simulink model "Helicopter_Model_Draft"  (R2024b)
settings: Solver=VariableStepAuto  StartTime=0.0  StopTime=100.0  RelTol=1e-3
StartFcn:
  | L1 = 3.13;
undefined symbols (not defined in the file): Earth, gravity, hRef, rad, rho, s, VRef, WGS84
libraries: slpidlib x9, simulink x2, aerolibfltsims x2, matrix_library x2, aerolibconvert2 x2, aerolibsim3d x2, aerolibatmos2 x1, aerolibtransform2 x1, shared6dof x1, sim3dlib x1
(part 2 of 2)

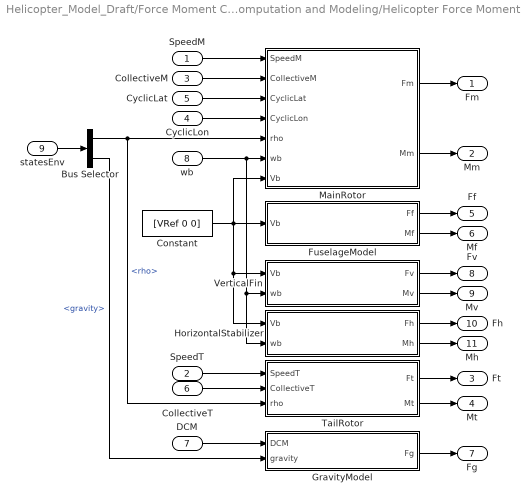
== system Helicopter_Model_Draft/Force Moment Computation and Modeling/Helicopter Force Moment Computation/ComputeForceandMoment ==
  SpeedM : Inport
  SpeedT : Inport  Port=2
  CollectiveM : Inport  Port=3
  CyclicLon : Inport  Port=4
  CyclicLat : Inport  Port=5
  CollectiveT : Inport  Port=6
  DCM : Inport  Port=7
  wb : Inport  Port=8
  statesEnv : Inport  Port=9
  Bus Selector : BusSelector  OutputSignals=rho,gravity
  Constant : Constant  Value=[VRef 0 0]
  FuselageModel : Subsystem
  GravityModel : Subsystem
  HorizontalStabilizer : MATLAB Function  TreatAsAtomicUnit=on
  MainRotor : Subsystem
  TailRotor : Subsystem
  VerticalFin : MATLAB Function  TreatAsAtomicUnit=on
  Fm : Outport
  Mm : Outport  Port=2
  Ft : Outport  Port=3
  Mt : Outport  Port=4
  Ff : Outport  Port=5
  Mf : Outport  Port=6
  Fg : Outport  Port=7
  Fv : Outport  Port=8
  Mv : Outport  Port=9
  Fh : Outport  Port=10
  Mh : Outport  Port=11
  wires:
  TailRotor/2(Mt) -> Mt/1
  MainRotor/1(Fm) -> Fm/1
  TailRotor/1(Ft) -> Ft/1
  FuselageModel/1(Ff) -> Ff/1
  MainRotor/2(Mm) -> Mm/1
  FuselageModel/2(Mf) -> Mf/1
  GravityModel/1(Fg) -> Fg/1
  Constant/1 -> HorizontalStabilizer/1(Vb), VerticalFin/1(Vb), MainRotor/7(Vb), FuselageModel/1(Vb)
  SpeedM/1 -> MainRotor/1(SpeedM)
  CollectiveT/1 -> TailRotor/2(CollectiveT)
  CollectiveM/1 -> MainRotor/2(CollectiveM)
  SpeedT/1 -> TailRotor/1(SpeedT)
  VerticalFin/1(Fv) -> Fv/1
  VerticalFin/2(Mv) -> Mv/1
  HorizontalStabilizer/1(Fh) -> Fh/1
  HorizontalStabilizer/2(Mh) -> Mh/1
  DCM/1 -> GravityModel/1(DCM)
  CyclicLon/1 -> MainRotor/4(CyclicLon)
  CyclicLat/1 -> MainRotor/3(CyclicLat)
  wb/1 -> HorizontalStabilizer/2(wb), VerticalFin/2(wb), MainRotor/6(wb)
  statesEnv/1 -> Bus Selector/1
  Bus Selector/1 -> MainRotor/5(rho), TailRotor/3(rho)  "<rho>"
  Bus Selector/2 -> GravityModel/2(gravity)  "<gravity>"

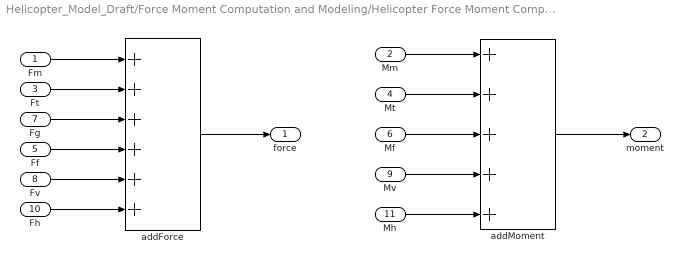
== system Helicopter_Model_Draft/Force Moment Computation and Modeling/Helicopter Force Moment Computation/ResultantForcesandMoments ==
  Fm : Inport
  Mm : Inport  Port=2
  Ft : Inport  Port=3
  Mt : Inport  Port=4
  Ff : Inport  Port=5
  Mf : Inport  Port=6
  Fg : Inport  Port=7
  Fv : Inport  Port=8
  Mv : Inport  Port=9
  Fh : Inport  Port=10
  Mh : Inport  Port=11
  addForce : Sum  Inputs=++++++
  addMoment : Sum  Inputs=+++++
  force : Outport
  moment : Outport  Port=2
  wires:
  Mt/1 -> addMoment/2
  Mf/1 -> addMoment/3
  addMoment/1 -> moment/1
  Ft/1 -> addForce/2
  Fm/1 -> addForce/1
  Fg/1 -> addForce/3
  Mm/1 -> addMoment/1
  Ff/1 -> addForce/4
  addForce/1 -> force/1
  Mh/1 -> addMoment/5
  Fh/1 -> addForce/6
  Fv/1 -> addForce/5
  Mv/1 -> addMoment/4

== system Helicopter_Model_Draft/Visualization/Variant Subsystem/Scope Visualization ==
  states : Inport
  Bus Selector : BusSelector  OutputSignals=Xe,angles,Vb,wb
  angle : Scope
  position : Scope
  rates : Scope
  velocity : Scope
  wires:
  states/1 -> Bus Selector/1
  Bus Selector/1 -> position/1  "<Xe>"
  Bus Selector/4 -> rates/1  "<wb>"
  Bus Selector/3 -> velocity/1  "<Vb>"
  Bus Selector/2 -> angle/1  "<angles>"

== system Helicopter_Model_Draft/Visualization/Variant Subsystem/Simulink 3D Animation ==
  states : Inport
  Add : Sum
  Bus Selector : BusSelector  OutputSignals=Xe,angles
  Constant10 : Constant  Value=[5000 0 -0.06]  VectorParams1D=off
  Simulation 3D Light Helicopter Pack : aerolibsim3d/Simulation 3D Light Helicopter Pack  Engine_T=off  Engine_R=off  Rotor1_T=off  Rotor1_R=on  Rotor2_T=off  Rotor2_R=on  Sensor1_T=off  Sensor1_R=off  Sensor2_T=off  Sensor2_R=off  GeoRadioButton=NED  AdjustForCesium=off  Heading0=90
  Simulation 3D Rotorcraft : aerolibsim3d/Simulation 3D Rotorcraft  Priority=-1  Mesh=Light helicopter  MeshPath=/MathWorksAerospaceContent/Vehicles/Rotorcraft/Helicopter/Mesh/SK_Helicopter.SK_Helicopter  MeshPathLight=/MathWorksAerospaceContent/Vehicles/Rotorcraft/LightHelicopter/Mesh/SK_LightHelicopter.SK_LightHelicopter  MeshPathMulti=/MathWorksAerospaceContent/Vehicles/Rotorcraft/Multirotor/Mesh/SK_Quadcopter.SK_Quadcopter  AircraftColor=Red  ActorName=SimulinkVehicle1  Translation=[5000 0 -0.06;zeros(5,3)]  Rotation=zeros(6, 3)  ScaleInputPort=Dialog  Scale=[1 1 1]  InitialScale=[1 1 1]  IsGHSensorEnabled=off  AreGHRaysVisible=off  IsOutputReshapeEnabled=off  GHRayLength=1524  GHBodyOffset=1.169  GHFrontTireRadius=0.196  GHLeftTireRadius=0.203  GHRightTireRadius=0.203  GHContactLocation1=[1.47 -1.04 1.169]  GHContactLocation2=[-1.24 -1.04 1.169]  GHContactLocation3=[-1.24 1.04 1.169]  GHContactLocation4=[1.47 1.04 1.169]  WoWSensorTolerance=0.05  LightsConfig=Automatic lights  LandingLightIntensity=300000  LandingLightConeAngle=15  LandingLightColor=[1 1 1]  HelicopterLeftLandingLightLocation=[0 0 0]  HelicopterLeftLandingLightOrientation=[0 0 0]  NoseLightIntensity=150000  NoseLightConeAngle=36  HelicopterNoseLightLocation=[0 0 0]  HelicopterNoseLightOrientation=[0 0 0]  NavLightIntensity=500  PositionLightIntensity=500  StrobeLightIntensity=5000  StrobeLightColor=[1 1 1]  StrobePeriod=1.5  StrobePulseWidth=6  BeaconLightIntensity=4000  BeaconLightColor=[1 0 0]  BeaconPeriod=1.5  BeaconPulseWidth=10  SampleTime=-1  ActorType=SimulinkVehicle  ID=1  aMode=0  ActorTag=SimulinkVehicle1
  Simulation 3D Scene Configuration : sim3dlib/Simulation 3D Scene Configuration  Priority=0  ProjectFormat=Default Scenes  SceneDesc=Airport  ProjectName=C:\Program Files\MATLAB\R2024b\toolbox\shared\sim3d_projects\automotive_project_windows\UE\WindowsNoEditor\VehicleSimulation.exe  ScenePath=/Game/Maps/HwStrght  EnableOpenDRIVE=off  vehTagList={'Scene Origin';'SimulinkVehicle1'}  vehTag=SimulinkVehicle1  FreeCameraInitialTranslation=[-6, 0, 2]  FreeCameraDefaultInitialTranslation=[-6, 0, 2]  FreeCameraInitialRotation=[0, -15, 0]  FreeCameraDefaultInitialRotation=[0, -15, 0]  OpVisEn=off  Ts=.02  EnableWindow=on  EnableRemoteAccess=off  EnableWeather=off  SunAzimuth=90  SunAltitude=40.0  EnableGeospatialSun=off  Latitude=0  Longitude=0  Date=2023-01-01  Time=10:30:00  GeoTimeZone=-5.0  SunDaylightSaving=off  wind=1  clouds=10  EnableVolumetricClouds=off  CloudCoverage=0  CloudAltitude=6  fog=0  rain=0  RaindropsEffect=off  SnowDensity=0  EnableGeospatial=off  UseTrueOrigin=off  OriginHeight=200  OriginLatitude=40.744652  OriginLongitude=-73.988864  MapStyle=Aerial  AdditionalAssetIDs=[]  UseAdvancedSunSky=off  SolarTime=11  TimeZone=-5  Day=21  Month=9  Year=2022  UseDaylightSavingTime=on  DSTStartDay=10  DSTStartMonth=3  DSTEndDay=3  DSTEndMonth=11  DSTSwitchHour=2  sensorTag=MainCamera1  sensorId=1  sensorName=MainCamera1  mountLoc=Origin  offsetFlag=off  tmountOffset=[0, 0, 0]  rmountOffset=[0, 0, 0]  HorizontalResolution=1280  VerticalResolution=720  HorizontalFOV=60  mountPoint=[0 0 0]  mountOrientation=[0 0 0]  aMode=0  ID=1  GeoTrigger=Inactive
  Subsystem : Subsystem
  speedM : Constant  Value=34
  speedT : Constant  Value=116
  wires:
  Bus Selector/2 -> Simulation 3D Light Helicopter Pack/2  "<angles>"
  states/1 -> Bus Selector/1
  speedT/1 -> Subsystem/2(SpeedT)
  speedM/1 -> Subsystem/1(SpeedM)
  Simulation 3D Light Helicopter Pack/1 -> Simulation 3D Rotorcraft/1
  Add/1 -> Simulation 3D Light Helicopter Pack/1
  Subsystem/2(Position Blade 2) -> Simulation 3D Light Helicopter Pack/4
  Constant10/1 -> Add/1
  Simulation 3D Light Helicopter Pack/2 -> Simulation 3D Rotorcraft/2
  Subsystem/1(Position Blade1) -> Simulation 3D Light Helicopter Pack/3
  Bus Selector/1 -> Add/2  "<Xe>"

== system Helicopter_Model_Draft/Attitude and Altitude Control/Reference Atttiude and Altitude Definition/Variant Subsystem/Hover ==
  Constant : Constant  Value=0
  ub : Outport
  wires:
  Constant/1 -> ub/1

== system Helicopter_Model_Draft/Attitude and Altitude Control/Reference Atttiude and Altitude Definition/Variant Subsystem/Level ==
  Vb : Inport
  Demux : Demux  Outputs=3
  Saturation1 : Saturate  UpperLimit=65  LowerLimit=0
  Sqrt : Sqrt
  Square1 : Math  Operator=square
  Square2 : Math  Operator=square
  Sum : Sum  Inputs=|+-
  Terminator : Terminator
  Terminator1 : Terminator
  V : Constant  Value=VRef
  ub : Outport
  wires:
  Square2/1 -> Sum/2
  Sum/1 -> Sqrt/1
  Square1/1 -> Sum/1
  Sqrt/1 -> Saturation1/1
  Vb/1 -> Demux/1
  Saturation1/1 -> ub/1
  Demux/3 -> Square2/1
  V/1 -> Square1/1
  Demux/1 -> Terminator/1
  Demux/2 -> Terminator1/1

== system Helicopter_Model_Draft/Force Moment Computation and Modeling/Helicopter Force Moment Computation/ComputeForceandMoment/FuselageModel ==
  Vb : Inport
  Abs : Abs  SaturateOnIntegerOverflow=off
  Abs1 : Abs  SaturateOnIntegerOverflow=off
  Abs2 : Abs  SaturateOnIntegerOverflow=off
  Demux : Demux  Outputs=3
  Fuselage Force Computation : Subsystem
  Fuselage Moment Computation : Subsystem
  Ff : Outport
  Mf : Outport  Port=2
  wires:
  Demux/1 -> Fuselage Force Computation/1(u), Fuselage Moment Computation/1(u), Abs/1
  Demux/2 -> Fuselage Force Computation/3(v), Abs1/1, Fuselage Moment Computation/3(v)
  Demux/3 -> Fuselage Moment Computation/4(w), Abs2/1, Fuselage Force Computation/5(w)
  Abs/1 -> Fuselage Moment Computation/2(absu), Fuselage Force Computation/2(absu)
  Vb/1 -> Demux/1
  Fuselage Moment Computation/1(Mf) -> Mf/1
  Abs1/1 -> Fuselage Force Computation/4(absv)
  Abs2/1 -> Fuselage Force Computation/6(absw)
  Fuselage Force Computation/1(Ff) -> Ff/1

== system Helicopter_Model_Draft/Force Moment Computation and Modeling/Helicopter Force Moment Computation/ComputeForceandMoment/GravityModel ==
  DCM : Inport
  gravity : Inport  Port=2
  Product : Product  Multiplication=Matrix(*)
  mass : Gain  Gain=2800
  Fg : Outport
  wires:
  mass/1 -> Product/2  "Fg_NED"
  gravity/1 -> mass/1
  Product/1 -> Fg/1
  DCM/1 -> Product/1

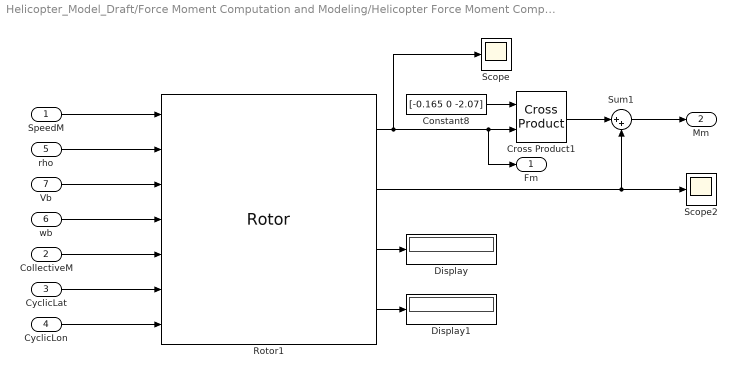
== system Helicopter_Model_Draft/Force Moment Computation and Modeling/Helicopter Force Moment Computation/ComputeForceandMoment/MainRotor ==
  SpeedM : Inport
  CollectiveM : Inport  Port=2
  CyclicLat : Inport  Port=3
  CyclicLon : Inport  Port=4
  rho : Inport  Port=5
  wb : Inport  Port=6
  Vb : Inport  Port=7
  Constant8 : Constant  Value=[-0.165 0 -2.07]  VectorParams1D=off
  Cross Product1 : matrix_library/Cross Product
  Display : Display
  Display1 : Display
  Rotor1 : Rotor  modelMode=With flap effects  controlInput=on  CTCQMode=Compute using BEMT  CT=0.0042  CQ=24e-5  CTout=on  radius=7.35  chord=0.53  cd0=0.009  gamma=10  thetaRoot=0.1493  thetaTwist=-0.1745
  Scope : Scope
  Scope2 : Scope
  Sum1 : Sum  Inputs=|++
  Fm : Outport
  Mm : Outport  Port=2
  wires:
  SpeedM/1 -> Rotor1/1
  Cross Product1/1 -> Sum1/1
  Constant8/1 -> Cross Product1/1
  Sum1/1 -> Mm/1
  Rotor1/2 -> Scope2/1, Sum1/2
  rho/1 -> Rotor1/2
  CollectiveM/1 -> Rotor1/5
  Rotor1/3 -> Display/1
  Rotor1/4 -> Display1/1
  Rotor1/1 -> Scope/1, Fm/1, Cross Product1/2
  wb/1 -> Rotor1/4
  Vb/1 -> Rotor1/3
  CyclicLat/1 -> Rotor1/6
  CyclicLon/1 -> Rotor1/7

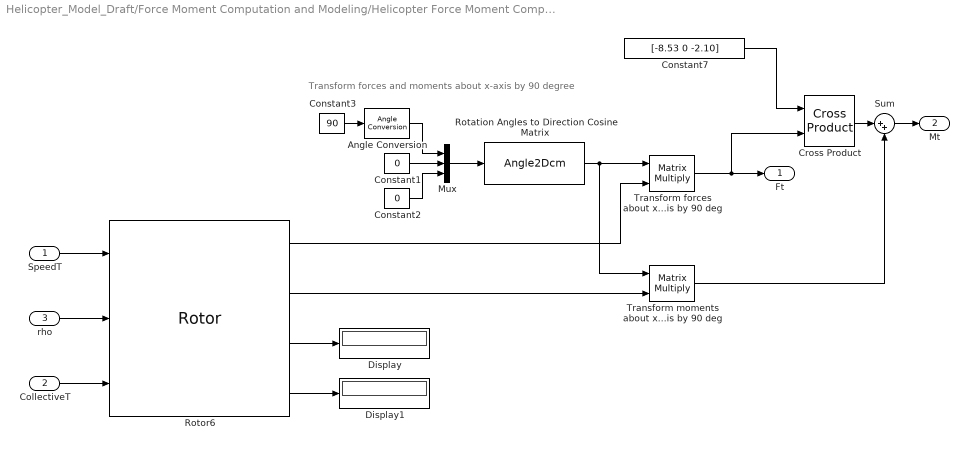
== system Helicopter_Model_Draft/Force Moment Computation and Modeling/Helicopter Force Moment Computation/ComputeForceandMoment/TailRotor ==
  note: Transform forces and moments about x-axis by 90 degree
  SpeedT : Inport
  CollectiveT : Inport  Port=2
  rho : Inport  Port=3
  Angle Conversion : aerolibconvert2/Angle Conversion  IU=deg  OU=rad
  Constant1 : Constant  Value=0
  Constant2 : Constant  Value=0
  Constant3 : Constant  Value=90
  Constant7 : Constant  Value=[-8.53 0 -2.10]  VectorParams1D=off
  Cross Product : matrix_library/Cross Product
  Display : Display
  Display1 : Display
  Mux : Mux  Inputs=3
  Rotation Angles to Direction Cosine Matrix : Angle2Dcm  rotationOrder=XYZ
      settings: AttributesFormatString=Rotation Order: %<rotationOrder>
  Rotor6 : Rotor  controlInput=on  CTCQMode=Compute using BEMT  CTout=on  radius=1.29  chord=0.2133  cd0=0.002  thetaRoot=0.015  thetaTwist=0
  Sum : Sum  Inputs=|++
  "Transform forces about x-axis by 90 deg " : Product  Multiplication=Matrix(*)
  Transform moments about x-axis by 90 deg : Product  Multiplication=Matrix(*)
  Ft : Outport
  Mt : Outport  Port=2
  wires:
  "Transform forces about x-axis by 90 deg "/1 -> Ft/1, Cross Product/2
  Rotor6/1 -> "Transform forces about x-axis by 90 deg "/2
  Transform moments about x-axis by 90 deg/1 -> Sum/2
  SpeedT/1 -> Rotor6/1
  Rotor6/2 -> Transform moments about x-axis by 90 deg/2
  Rotation Angles to Direction Cosine Matrix/1 -> "Transform forces about x-axis by 90 deg "/1, Transform moments about x-axis by 90 deg/1
  Cross Product/1 -> Sum/1
  Constant7/1 -> Cross Product/1
  Sum/1 -> Mt/1
  CollectiveT/1 -> Rotor6/3
  rho/1 -> Rotor6/2
  Rotor6/4 -> Display1/1
  Rotor6/3 -> Display/1
  Angle Conversion/1 -> Mux/1
  Mux/1 -> Rotation Angles to Direction Cosine Matrix/1
  Constant3/1 -> Angle Conversion/1
  Constant1/1 -> Mux/2
  Constant2/1 -> Mux/3

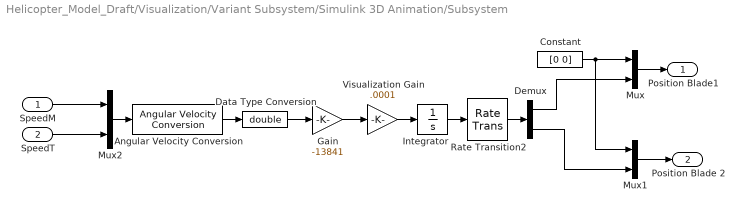
== system Helicopter_Model_Draft/Visualization/Variant Subsystem/Simulink 3D Animation/Subsystem ==
  SpeedM : Inport
  SpeedT : Inport  Port=2
  Angular Velocity Conversion : aerolibconvert2/Angular Velocity Conversion  IU=rad/s  OU=rpm
  Constant : Constant  Value=[0 0]  VectorParams1D=off
  Data Type Conversion : DataTypeConversion  OutDataTypeStr=double  SaturateOnIntegerOverflow=off  RndMeth=Floor
  Demux : Demux  Outputs=2
  Gain : Gain  Gain=-13841
  Integrator : Integrator  InitialCondition="[.1  .1]"  WrapState=on  WrappedStateUpperValue=2*pi  WrappedStateLowerValue=-2*pi
  Mux : Mux  Inputs=2
  Mux1 : Mux  Inputs=2
  Mux2 : Mux  Inputs=2
  Rate Transition2 : RateTransition
  Visualization Gain : Gain  Gain=.0001
  Position Blade1 : Outport  VectorParamsAs1DForOutWhenUnconnected=off
  Position Blade 2 : Outport  Port=2  VectorParamsAs1DForOutWhenUnconnected=off
  wires:
  Demux/2 -> Mux1/2
  Visualization Gain/1 -> Integrator/1
  Constant/1 -> Mux1/1, Mux/1
  Mux1/1 -> Position Blade 2/1
  Data Type Conversion/1 -> Gain/1
  Integrator/1 -> Rate Transition2/1
  Mux/1 -> Position Blade1/1
  Gain/1 -> Visualization Gain/1
  Demux/1 -> Mux/2
  Mux2/1 -> Angular Velocity Conversion/1
  Rate Transition2/1 -> Demux/1
  SpeedM/1 -> Mux2/1
  SpeedT/1 -> Mux2/2
  Angular Velocity Conversion/1 -> Data Type Conversion/1

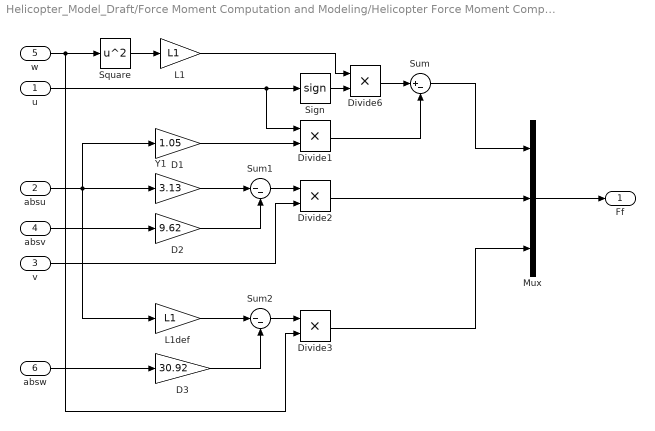
== system Helicopter_Model_Draft/Force Moment Computation and Modeling/Helicopter Force Moment Computation/ComputeForceandMoment/FuselageModel/Fuselage Force Computation ==
  u : Inport
  absu : Inport  Port=2
  v : Inport  Port=3
  absv : Inport  Port=4
  w : Inport  Port=5
  absw : Inport  Port=6
  D1 : Gain  Gain=1.05
  D2 : Gain  Gain=9.62
  D3 : Gain  Gain=30.92
  Divide{1..3,6} (4 alike) : Product  Inputs=**
  L1 : Gain  Gain=L1
  L1def : Gain  Gain=L1
  Mux : Mux  Inputs=3
  Sign : Signum
  Square : Math  Operator=square
  Sum : Sum  Inputs=|+-
  Sum1 : Sum  Inputs=|--
  Sum2 : Sum  Inputs=|--
  Y1 : Gain  Gain=3.13
  Ff : Outport
  wires:
  Sign/1 -> Divide6/2
  D2/1 -> Sum1/2
  Sum1/1 -> Divide2/1
  Divide6/1 -> Sum/1
  Divide2/1 -> Mux/2
  D3/1 -> Sum2/2
  u/1 -> Divide1/1, Sign/1
  L1def/1 -> Sum2/1
  Divide1/1 -> Sum/2
  Y1/1 -> Sum1/1
  absv/1 -> D2/1
  Square/1 -> L1/1
  L1/1 -> Divide6/1
  Sum/1 -> Mux/1
  Divide3/1 -> Mux/3
  Sum2/1 -> Divide3/1
  v/1 -> Divide2/2
  absw/1 -> D3/1
  Mux/1 -> Ff/1
  w/1 -> Square/1, Divide3/2
  absu/1 -> D1/1, Y1/1, L1def/1
  D1/1 -> Divide1/2

== system Helicopter_Model_Draft/Force Moment Computation and Modeling/Helicopter Force Moment Computation/ComputeForceandMoment/FuselageModel/Fuselage Moment Computation ==
  u : Inport
  absu : Inport  Port=2
  v : Inport  Port=3
  w : Inport  Port=4
  Constant : Constant  Value=0
  Divide4 : Product  Inputs=**
  Divide5 : Product  Inputs=**
  M1 : Gain  Gain=13.95
  Mux1 : Mux  Inputs=3
  N1 : Gain  Gain=13.95
  Unary Minus : UnaryMinus
  Mf : Outport
  wires:
  u/1 -> Divide5/1
  M1/1 -> Divide4/2
  N1/1 -> Unary Minus/1
  Mux1/1 -> Mf/1
  Divide5/1 -> Mux1/3
  Constant/1 -> Mux1/1
  v/1 -> N1/1
  Unary Minus/1 -> Divide5/2
  Divide4/1 -> Mux1/2
  w/1 -> M1/1
  absu/1 -> Divide4/1

== matlab function Helicopter_Model_Draft/Force Moment Computation and Modeling/Helicopter Force Moment Computation/ComputeForceandMoment/VerticalFin ==
  data: Vb input; Fv output; wb input; Mv output
function [Fv,Mv] = VerticalFin(Vb,wb)
lvf = 7.62;
K1 = 1.40;
F1 = 0.77;
vf = -Vb(2)+lvf*wb(3);
Yv = K1*vf*Vb(1)+F1*vf*abs(vf);
Fv = [0 Yv 0];
Mv = [0 0 -Yv*lvf];

== matlab function Helicopter_Model_Draft/Force Moment Computation and Modeling/Helicopter Force Moment Computation/ComputeForceandMoment/HorizontalStabilizer ==
  data: Vb input; Fh output; wb input; Mh output
function [Fh,Mh] = HorizontalStabilizer(Vb,wb)
lhs = 6;
H1 = 1.48;
H4 = 0.40;
wh = Vb(3)+lhs*wb(2);
Zh = -H1*wh*Vb(1) - H4*wh*abs(wh);
Fh = [0 0 Zh];
Mh = [0 Zh*lhs 0];
